simulink model "excercise1_bd_ex4"  (R2023b)
settings: Solver=VariableStepAuto  StartTime=0.0  StopTime=0.3  RelTol=1e-3
model workspace (MATLAB code in the model file):
  | R = 200;
  | C = 10*10^(-6);
settings Model: Creator=elliot  LastModifiedBy=elliot

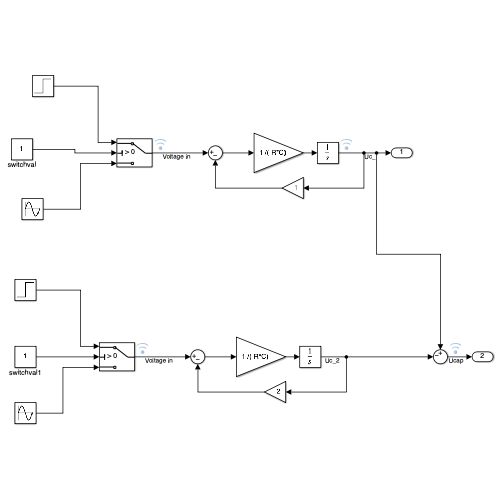
[thumbnail: Simulink's stored preview of the top-level diagram]
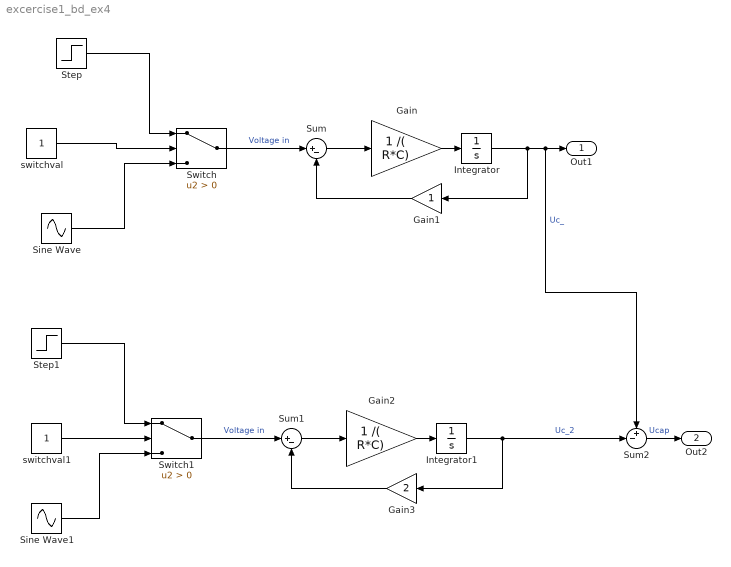
== system excercise1_bd_ex4 ==
  Gain : Gain  Gain=1 /( R*C)
  Gain1 : Gain
  Gain2 : Gain  Gain=1 /( R*C)
  Gain3 : Gain  Gain=2
  Integrator : Integrator
  Integrator1 : Integrator
  Sine Wave : Sin  Frequency=10  SampleTime=0
  Sine Wave1 : Sin  Frequency=10  SampleTime=0
  Step : Step  Time=0  After=12  SampleTime=0
  Step1 : Step  Time=0.2  After=12  SampleTime=0
  Sum : Sum  Inputs=|+-
  Sum1 : Sum  Inputs=|+-
  Sum2 : Sum  Inputs=+-|
  Switch : Switch  Criteria=u2 > Threshold  SaturateOnIntegerOverflow=off  InputSameDT=off
  Switch1 : Switch  Criteria=u2 > Threshold  SaturateOnIntegerOverflow=off  InputSameDT=off
  switchval : Constant
  switchval1 : Constant
  Out1 : Outport
  Out2 : Outport  Port=2
  wires:
  Switch/1 -> Sum/1  "Voltage in"
  Step/1 -> Switch/1
  Sine Wave/1 -> Switch/3
  switchval/1 -> Switch/2
  Gain1/1 -> Sum/2
  Sum/1 -> Gain/1
  Gain/1 -> Integrator/1
  Integrator/1 -> Gain1/1, Sum2/1, Out1/1  "Uc_"
  Sum1/1 -> Gain2/1
  Switch1/1 -> Sum1/1  "Voltage in"
  Gain2/1 -> Integrator1/1
  Sine Wave1/1 -> Switch1/3
  switchval1/1 -> Switch1/2
  Step1/1 -> Switch1/1
  Gain3/1 -> Sum1/2
  Integrator1/1 -> Sum2/2, Gain3/1  "Uc_2"
  Sum2/1 -> Out2/1  "Ucap"
